simulink model "AboveBelowThresholdMultiSiteDetector"  (R2016b)
settings: Solver=FixedStepDiscrete  StartTime=0.0  StopTime=inf  FixedStep=sCoreParams.core.stepPeriod  RelTol=1e-3
undefined symbols (not defined in the file): sCoreParams, sCoreParams_stimulator_stimChannelLower, sCoreParams_stimulator_stimChannelUpper
libraries: dspstat3 x2, simulink x1, dspswit3 x1, commutil2 x1, dspindex x1
settings Model: DataTypeOverride=Double  MinMaxOverflowLogging=ForceOff  Creator=anish  LastModifiedBy=Rina
settings SolverCC: EnableConcurrentExecution=on
settings DataIOCC: SaveFormat=StructureWithTime  SignalLoggingSaveFormat=ModelDataLogs  SaveOutput=off  SignalLogging=off  DSMLogging=off  SaveTime=off
settings OptimizationCC: BlockReduction=off  ConditionallyExecuteInputs=off  DefaultParameterBehavior=Inlined  OptimizeBlockIOStorage=off  BufferReuse=off  GlobalBufferReuse=off  ExpressionFolding=off  LocalBlockOutputs=off  LifeSpan=inf
settings DebuggingCC: SignalRangeChecking=error  SaveWithParameterizedLinksMsg=none  MultiTaskDSMMsg=warning  MultiTaskCondExecSysMsg=none  AllowSymbolicDim=off  ModelReferenceSymbolNameMessage=none  StateNameClashWarn=warning  SFUnexpectedBacktrackingDiag=warning  SFNoUnconditionalDefaultTransitionDiag=warning  SFExecutionAtInitializationDiag=none
settings HardwareCC: ProdBitPerPointer=32  ProdBitPerSizeT=32  ProdBitPerPtrDiffT=32  ProdLargestAtomicFloat=None  ProdWordSize=32  ProdLongLongMode=on  ProdHWDeviceType=Generic->32-bit x86 compatible  TargetBitPerPointer=64  TargetLargestAtomicFloat=Float  TargetLongLongMode=on  TargetIntDivRoundTo=Zero  TargetEndianess=LittleEndian  TargetWordSize=64  TargetHWDeviceType=Intel->x86-64 (Windows64)
settings ModelReferenceCC: UpdateModelReferenceTargets=Force  ModelReferenceNumInstancesAllowed=Single  ModelReferencePassRootInputsByReference=off
settings RTWCC: SystemTargetFile=slrt.tlc  TemplateMakefile=slrt_default_tmf  Description=Simulink Real-Time  BuildConfiguration=Faster Runs  RTWCompilerOptimization=on
settings TargetCC: CodeReplacementLibrary=XPC_BLAS  ParMdlRefBuildCompliant=on  ConcurrentExecutionCompliant=on  GeneratePreprocessorConditionals=Use local settings  MatFileLogging=on  MATLABClassNameForMDSCustomization=xpcAperiodicCustomization
settings ConfigComp: CovMetricSettings=dw  CovHtmlReporting=on  CovSaveCumulativeToWorkspaceVar=on  CovSaveSingleToWorkspaceVar=on  CovExternalEMLEnable=off  CovSFcnEnable=off

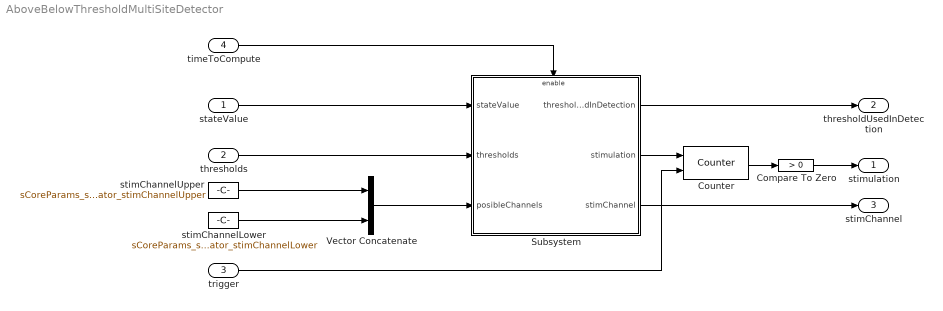
== system AboveBelowThresholdMultiSiteDetector ==
  stateValue : Inport  PortDimensions=1  SampleTime=sCoreParams.core.stepPeriod
  thresholds : Inport  Port=2  PortDimensions=[1 2]  SampleTime=sCoreParams.core.stepPeriod
  trigger : Inport  Port=3  OutDataTypeStr=boolean  SampleTime=sCoreParams.core.stepPeriod
  timeToCompute : Inport  Port=4  OutDataTypeStr=boolean  SampleTime=sCoreParams.core.stepPeriod
  Compare To Zero : simulink/Logic and Bit Operations/Compare To Zero  relop=>  OutDataTypeStr=boolean
  Counter : dspswit3/Counter  Direction=Up  CountEvent=Non-zero sample  CounterSize=16 bits  MaxCount=sCoreParams.decoders.txDetector.detectionDurationSamples  InitialCount=0  Output=Count  HitValue=sCoreParams.decoders.txDetector.detectionDurationSamples  ResetInput=on  SamplesPerFrame=1  Ts=sCoreParams.core.stepPeriod  CntDtype=int32  HitDtype=Logical
  Subsystem : Subsystem
  Vector Concatenate : Concatenate  Mode=Multidimensional array
  stimChannelLower : Constant  Value=sCoreParams_stimulator_stimChannelLower  VectorParams1D=off
  stimChannelUpper : Constant  Value=sCoreParams_stimulator_stimChannelUpper  VectorParams1D=off
  stimulation : Outport
  thresholdUsedInDetection : Outport  Port=2
  stimChannel : Outport  Port=3  OutDataTypeStr=int32
  wires:
  thresholds/1 -> Subsystem/2(thresholds)
  stimChannelUpper/1 -> Vector Concatenate/1
  Subsystem/1(thresholdUsedInDetection) -> thresholdUsedInDetection/1
  Subsystem/3(stimChannel) -> stimChannel/1
  stateValue/1 -> Subsystem/1(stateValue)
  Counter/1 -> Compare To Zero/1
  Compare To Zero/1 -> stimulation/1
  Subsystem/2(stimulation) -> Counter/1
  trigger/1 -> Counter/2
  timeToCompute/1 -> Subsystem/Enable
  Vector Concatenate/1 -> Subsystem/3(posibleChannels)
  stimChannelLower/1 -> Vector Concatenate/2

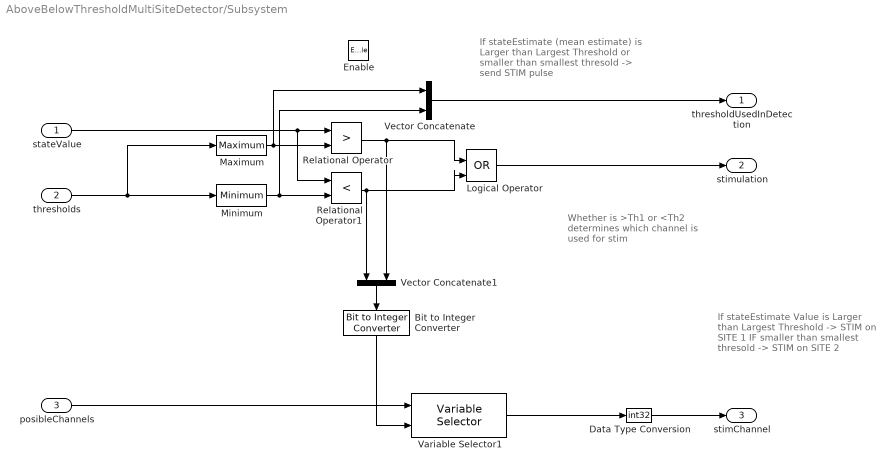
== system AboveBelowThresholdMultiSiteDetector/Subsystem ==
  note: Whether is >Th1 or <Th2
      | determines which channel
      |  is used for stim
  note: If stateEstimate (mean estimate)
      | is Larger than Largest Threshold
      | or
      | smaller than smallest thresold
      | -> send STIM pulse
  note: If stateEstimate Value
      | is Larger than Largest Threshold
      | -> STIM on SITE 1
      | IF smaller than smallest thresold
      | ->  STIM on SITE 2
  stateValue : Inport  PortDimensions=1
  thresholds : Inport  Port=2  PortDimensions=[1 2]
  posibleChannels : Inport  Port=3
  Enable : EnablePort
  Bit to Integer Converter : commutil2/Bit to Integer Converter  nbits=2  bitOrder=MSB first  signedOutputValues=Unsigned  outDtype=Inherit via internal rule  outDtypeSigned=Inherit via internal rule
  Data Type Conversion : DataTypeConversion  OutDataTypeStr=int32
  Logical Operator : Logic  Operator=OR  IconShape=distinctive  AllPortsSameDT=off  OutDataTypeStr=boolean
  Maximum : dspstat3/Maximum  operation=maximum  fcn=Value  indexBase=One  operateOver=Entire input  Dimension=2  InputProcessing=Columns as channels (frame based)  reset=None  roiEnable=off  roiType=Rectangles  roiPortion=Entire ROI  roiOutput=Individual statistics for each ROI  roiFlag=off  roundingMode=Floor  overflowMode=off  accumDataTypeStr=Inherit: Same as product output  accumLastDataTypeStr=Inherit: Same as product output
  Minimum : dspstat3/Minimum  operation=minimum  fcn=Value  indexBase=One  operateOver=Entire input  Dimension=1  InputProcessing=Columns as channels (frame based)  reset=None  roiEnable=off  roiType=Rectangles  roiPortion=Entire ROI  roiOutput=Individual statistics for each ROI  roiFlag=off  roundingMode=Floor  overflowMode=off
  Relational Operator : RelationalOperator  Operator=>  OutDataTypeStr=boolean  RndMeth=Simplest
  Relational Operator1 : RelationalOperator  Operator=<  OutDataTypeStr=boolean  RndMeth=Simplest
  Variable Selector1 : dspindex/Variable Selector  NumInputs=1  rowsOrCols=Rows  IdxMode=Variable  Elements=[1 3]  ZerOneIdxMode=One-based  errmode=Clip Index  FillMode=on  FillValues=0
  Vector Concatenate : Concatenate
  Vector Concatenate1 : Concatenate
  thresholdUsedInDetection : Outport
  stimulation : Outport  Port=2  OutputWhenDisabled=reset  InitialOutput=0
  stimChannel : Outport  Port=3
  wires:
  thresholds/1 -> Maximum/1, Minimum/1
  Vector Concatenate/1 -> thresholdUsedInDetection/1
  Logical Operator/1 -> stimulation/1
  Bit to Integer Converter/1 -> Variable Selector1/2
  Relational Operator/1 -> Vector Concatenate1/2, Logical Operator/1
  Variable Selector1/1 -> Data Type Conversion/1
  Vector Concatenate1/1 -> Bit to Integer Converter/1
  Relational Operator1/1 -> Vector Concatenate1/1, Logical Operator/2
  Data Type Conversion/1 -> stimChannel/1
  posibleChannels/1 -> Variable Selector1/1
  stateValue/1 -> Relational Operator1/1, Relational Operator/1
  Maximum/1 -> Relational Operator/2, Vector Concatenate/1
  Minimum/1 -> Vector Concatenate/2, Relational Operator1/2
